simulink model "senario_1"  (R2020a)
settings: Solver=VariableStepAuto  StartTime=0.0  StopTime=10.0  RelTol=1e-3
libraries: fuzblock x2, simulink x1
settings Model: Creator=MANOS  LastModifiedBy=MANOS

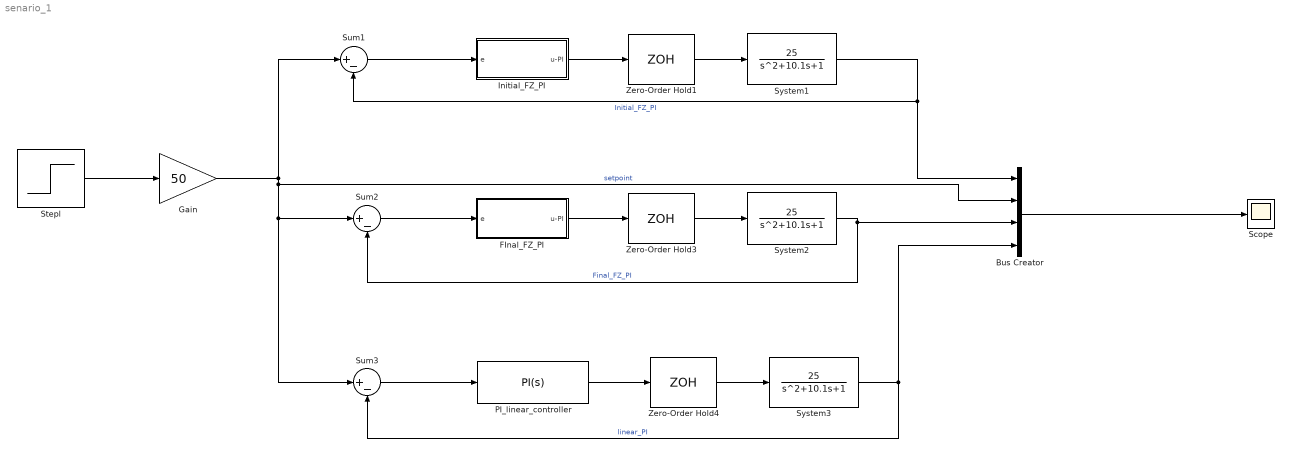
== system senario_1 ==
  Bus Creator : BusCreator  Inputs=4
  FInal_FZ_PI : Subsystem
  Gain : Gain  Gain=50
  Initial_FZ_PI : Subsystem
  PI_linear_controller : simulink/Continuous/PID Controller  Controller=PI  Form=Parallel  TimeDomain=Continuous-time  UseExternalTs=off  SampleTime=-1  IntegratorMethod=Forward Euler  FilterMethod=Forward Euler  ControllerParametersSource=internal  P=1.262  I=0.36598  D=0.02  UseFilter=on  N=20  TunerSelectOption=Transfer Function Based (PID Tuner App)  InitialConditionSource=internal  InitialConditionForIntegrator=0  InitialConditionForFilter=0  DifferentiatorICPrevScaledInput=0  ExternalReset=none  TrackingMode=off  Kt=1  LimitOutput=off  UpperSaturationLimit=inf  LowerSaturationLimit=-inf  LinearizeAsGain=on  AntiWindupMode=none  Kb=1  POutMin=[]  POutMax=[]  IOutMin=[]  IOutMax=[]  DOutMin=[]  DOutMax=[]  NOutMin=[]  NOutMax=[]  SumOutMin=[]  SumOutMax=[]  SaturationOutMin=[]  SaturationOutMax=[]  PParamMin=[]  PParamMax=[]  IParamMin=[]  IParamMax=[]  DParamMin=[]  DParamMax=[]  NParamMin=[]  NParamMax=[]  KbParamMin=[]  KbParamMax=[]  KtParamMin=[]  KtParamMax=[]  KbOutMin=[]  KbOutMax=[]  KtOutMin=[]  KtOutMax=[]  IntegratorOutMin=[]  IntegratorOutMax=[]  FilterOutMin=[]  FilterOutMax=[]  SumI1OutMin=[]  SumI1OutMax=[]  SumI2OutMin=[]  SumI2OutMax=[]  SumI3OutMin=[]  SumI3OutMax=[]  SumI4OutMin=[]  SumI4OutMax=[]  SumDOutMin=[]  SumDOutMax=[]  DifferentiatorOutMin=[]  DifferentiatorOutMax=[]  FilterDiffOutCoefMin=[]  FilterDiffOutCoefMax=[]  ReciprocalOutMin=[]  ReciprocalOutMax=[]  SumDenOutMin=[]  SumDenOutMax=[]  SumNumOutMin=[]  SumNumOutMax=[]  DivideOutMin=[]  DivideOutMax=[]  UdiffTsProdOutMin=[]  UdiffTsProdOutMax=[]  NTsProdOutMin=[]  NTsProdOutMax=[]  UintegralTsProdOutMin=[]  UintegralTsProdOutMax=[]  UngainTsProdOutMin=[]  UngainTsProdOutMax=[]  IntegratorContinuousStateAttributes=''  IntegratorStateMustResolveToSignalObject=off  IntegratorRTWStateStorageClass=Auto  FilterContinuousStateAttributes=''  FilterStateMustResolveToSignalObject=off  FilterRTWStateStorageClass=Auto  ParallelPVariant=InternalParameters  IdealPVariant=Disabled  IVariant=InternalParameters  DVariant=Disabled  IntegratorVariant=Continuous  SatVariant=Disabled  AWVariant=Passthrough  PCopyVariant=Disabled  TRVariant=Disabled  FdbkBlocksVariant=Forward  IdealPFdbkVariant=Disabled  SatFdbkVariant=Disabled  DerivativeFilterVariant=Disabled  NVariant=Disabled  NCopyVariant=Disabled_SignalSpec  FilterICVariant=Disabled  IntegratorICVariant=InternalICs  ExternalResetVariant=Disabled  TRSumVariant=Passthrough  SumFdbkVariant=Disabled  SumVariant=Sum_PI  TsampFilterVariant=InternalTs  TsampNgainVariant=Passthrough  TsampIntegralVariant=Passthrough
  Scope : Scope
  Stepl : Step  Time=0  SampleTime=0.01
  Sum1 : Sum  Inputs=|+-
  Sum2 : Sum  Inputs=|+-
  Sum3 : Sum  Inputs=|+-
  System1 : TransferFcn  Numerator=[25]  Denominator=[1 10.1 1]
  System2 : TransferFcn  Numerator=[25]  Denominator=[1 10.1 1]
  System3 : TransferFcn  Numerator=[25]  Denominator=[1 10.1 1]
  Zero-Order Hold1 : ZeroOrderHold  SampleTime=-1
  Zero-Order Hold3 : ZeroOrderHold  SampleTime=-1
  Zero-Order Hold4 : ZeroOrderHold  SampleTime=-1
  wires:
  Stepl/1 -> Gain/1
  Gain/1 -> Sum3/1, Sum2/1, Bus Creator/2, Sum1/1  "setpoint"
  Sum1/1 -> Initial_FZ_PI/1(e)
  Sum2/1 -> FInal_FZ_PI/1(e)
  Sum3/1 -> PI_linear_controller/1
  FInal_FZ_PI/1(u-PI) -> Zero-Order Hold3/1
  System2/1 -> Bus Creator/3, Sum2/2  "Final_FZ_PI"
  Zero-Order Hold1/1 -> System1/1
  PI_linear_controller/1 -> Zero-Order Hold4/1
  Initial_FZ_PI/1(u-PI) -> Zero-Order Hold1/1
  Zero-Order Hold4/1 -> System3/1
  Zero-Order Hold3/1 -> System2/1
  System1/1 -> Bus Creator/1, Sum1/2  "Initial_FZ_PI"
  System3/1 -> Bus Creator/4, Sum3/2  "linear_PI"
  Bus Creator/1 -> Scope/1

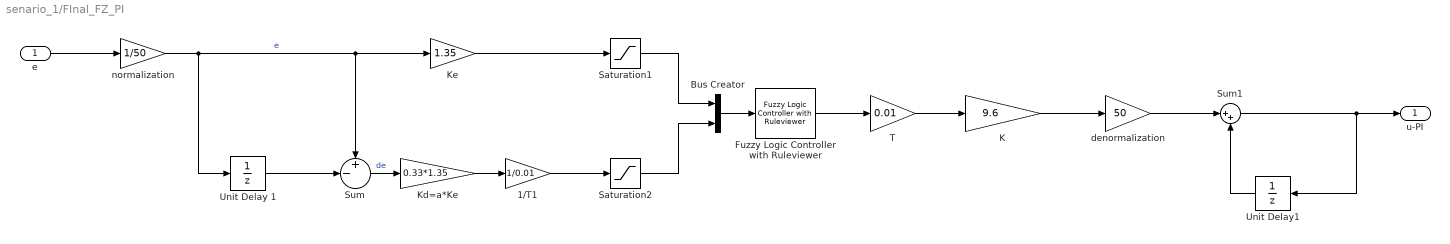
== system senario_1/FInal_FZ_PI ==
  e : Inport
  1/T1 : Gain  Gain=1/0.01
  Bus Creator : BusCreator  Inputs=2
  Fuzzy Logic Controller with Ruleviewer : fuzblock/Fuzzy Logic  Controller  with Ruleviewer  fismatrix=FLC  Ts=2
  K : Gain  Gain=9.6
  Kd=a*Ke : Gain  Gain=0.33*1.35
  Ke : Gain  Gain=1.35
  Saturation1 : Saturate  UpperLimit=1  LowerLimit=-1
  Saturation2 : Saturate  UpperLimit=1  LowerLimit=-1
  Sum : Sum  Inputs=+-|
  Sum1 : Sum  Inputs=|++
  T : Gain  Gain=0.01
  Unit Delay 1 : UnitDelay  SampleTime=-1  HasFrameUpgradeWarning=on
  Unit Delay1 : UnitDelay  SampleTime=-1  HasFrameUpgradeWarning=on
  denormalization : Gain  Gain=50
  normalization : Gain  Gain=1/50
  u-PI : Outport
  wires:
  denormalization/1 -> Sum1/1
  Sum1/1 -> u-PI/1, Unit Delay1/1
  K/1 -> denormalization/1
  T/1 -> K/1
  Bus Creator/1 -> Fuzzy Logic Controller with Ruleviewer/1
  Ke/1 -> Saturation1/1
  normalization/1 -> Ke/1, Sum/1, Unit Delay 1/1  "e"
  Fuzzy Logic Controller with Ruleviewer/1 -> T/1
  1/T1/1 -> Saturation2/1
  Unit Delay1/1 -> Sum1/2
  Sum/1 -> Kd=a*Ke/1  "de"
  Kd=a*Ke/1 -> 1/T1/1
  Saturation2/1 -> Bus Creator/2
  Unit Delay 1/1 -> Sum/2
  e/1 -> normalization/1
  Saturation1/1 -> Bus Creator/1

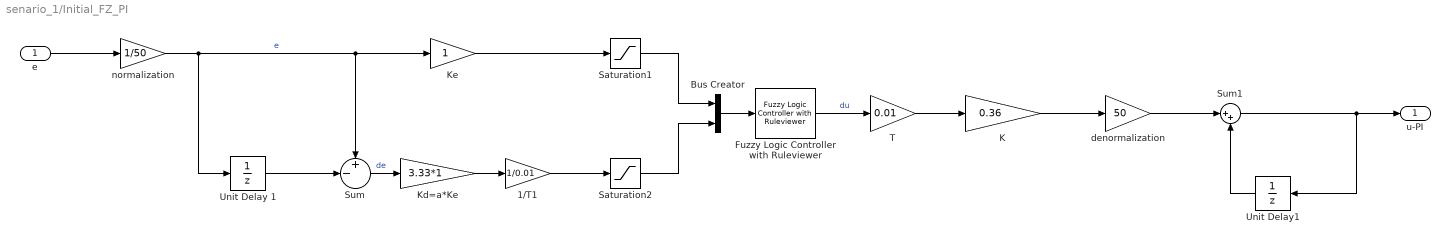
== system senario_1/Initial_FZ_PI ==
  e : Inport
  1/T1 : Gain  Gain=1/0.01
  Bus Creator : BusCreator  Inputs=2
  Fuzzy Logic Controller with Ruleviewer : fuzblock/Fuzzy Logic  Controller  with Ruleviewer  fismatrix=FLC  Ts=2
  K : Gain  Gain=0.36
  Kd=a*Ke : Gain  Gain=3.33*1
  Ke : Gain
  Saturation1 : Saturate  UpperLimit=1  LowerLimit=-1
  Saturation2 : Saturate  UpperLimit=1  LowerLimit=-1
  Sum : Sum  Inputs=+-|
  Sum1 : Sum  Inputs=|++
  T : Gain  Gain=0.01
  Unit Delay 1 : UnitDelay  SampleTime=-1  HasFrameUpgradeWarning=on
  Unit Delay1 : UnitDelay  SampleTime=-1  HasFrameUpgradeWarning=on
  denormalization : Gain  Gain=50
  normalization : Gain  Gain=1/50
  u-PI : Outport
  wires:
  Unit Delay 1/1 -> Sum/2
  normalization/1 -> Ke/1, Sum/1, Unit Delay 1/1  "e"
  e/1 -> normalization/1
  Sum/1 -> Kd=a*Ke/1  "de"
  Kd=a*Ke/1 -> 1/T1/1
  Ke/1 -> Saturation1/1
  1/T1/1 -> Saturation2/1
  Saturation1/1 -> Bus Creator/1
  Saturation2/1 -> Bus Creator/2
  Bus Creator/1 -> Fuzzy Logic Controller with Ruleviewer/1
  Fuzzy Logic Controller with Ruleviewer/1 -> T/1  "du"
  T/1 -> K/1
  K/1 -> denormalization/1
  Sum1/1 -> u-PI/1, Unit Delay1/1
  Unit Delay1/1 -> Sum1/2
  denormalization/1 -> Sum1/1
